simulink model "SeparateMotorModel"  (R2015b)
settings: Solver=VariableStepAuto  StartTime=0.0  StopTime=10.0  RelTol=1e-3
undefined symbols (not defined in the file): Initial, Motor, Uav
libraries: QuaternionLibrary x1, simulink_extras x1
settings Model: Creator=jban039  LastModifiedBy=jban039

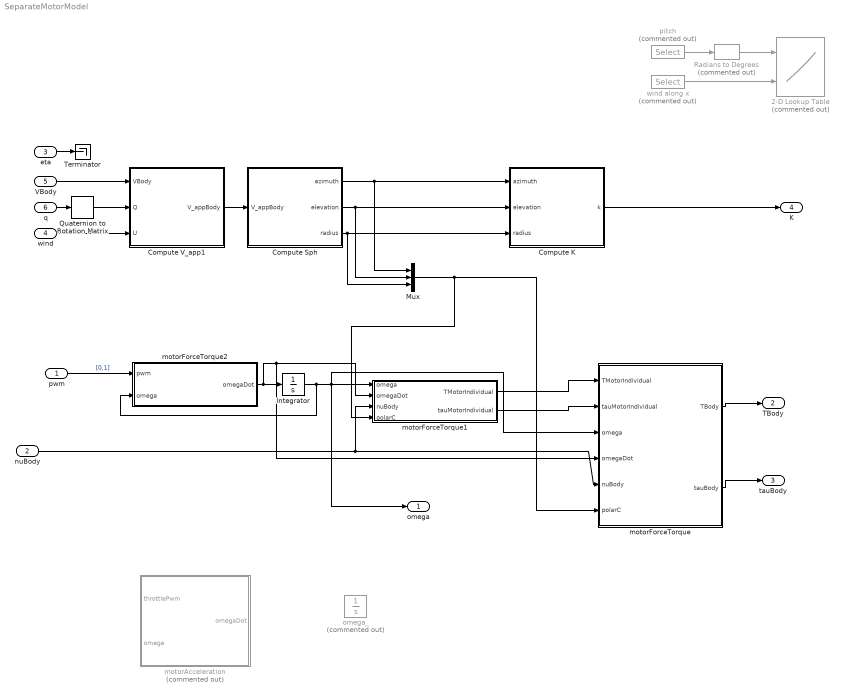
== system SeparateMotorModel ==
  pwm : Inport  PortDimensions=Uav.N_ROTORS
  nuBody : Inport  Port=2
  eta : Inport  Port=3  PortDimensions=3
  wind : Inport  Port=4  PortDimensions=3
  VBody : Inport  Port=5  PortDimensions=3
  q : Inport  Port=6  PortDimensions=4
  2-D Lookup Table : Lookup_n-D  Commented=on  BreakpointsForDimension1=[0,2.890909,6.009259676377,9.296238414,12.27875]  BreakpointsForDimension2=[0,10,20]  Table=reshape([9.55641004221352e-06,1.00990801427108e-05,1.28091919414946e-05,1.45562427543497e-05,1.63017404112369e-05,1.00884339028815e-05,1.06718323589317e-05,1.12577089455794e-05,1.21229824131359e-05,1.24606394544993e-05,9.47230336229989e-06,9.71233115660863e-06,9.65341998978562e-06,9.60249125674676e-06,8.92828582195144e-06],5,3)  InternalRulePriority=Speed  RndMeth=Simplest  InputSameDT=on
  Compute K : MATLAB Function  TreatAsAtomicUnit=on
  Compute Sph : MATLAB Function  TreatAsAtomicUnit=on
  Compute V_app1 : MATLAB Function  TreatAsAtomicUnit=on
  Integrator : Integrator
  Mux : Mux  Inputs=3
  Quaternion to Rotation Matrix : QuaternionLibrary/Quaternion to Rotation Matrix
  Radians to Degrees : simulink_extras/Transformations/Radians to Degrees  Commented=on
  Terminator : Terminator
  motorAcceleration : MATLAB Function  Commented=on  TreatAsAtomicUnit=on
  motorForceTorque : MATLAB Function  TreatAsAtomicUnit=on
  motorForceTorque1 : MATLAB Function  TreatAsAtomicUnit=on
  motorForceTorque2 : MATLAB Function  TreatAsAtomicUnit=on
  omega_ : Integrator  Commented=on  InitialCondition=Initial.OMEGA
  pitch : Selector  Commented=on  InputPortWidth=3  IndexOptions=Index vector (dialog)  Indices=[2]  OutputSizes=1
  wind along x : Selector  Commented=on  InputPortWidth=3  IndexOptions=Index vector (dialog)  Indices=[1]  OutputSizes=1
  omega : Outport
  TBody : Outport  Port=2
  tauBody : Outport  Port=3
  K : Outport  Port=4
  wires:
  motorForceTorque/2(tauBody) -> tauBody/1
  motorForceTorque/1(TBody) -> TBody/1
  pwm/1 -> motorForceTorque2/1(pwm)  "[0,1]"
  wind along x/1 -> 2-D Lookup Table/2
  pitch/1 -> Radians to Degrees/1
  Compute K/1(k) -> K/1
  Radians to Degrees/1 -> 2-D Lookup Table/1
  Quaternion to Rotation Matrix/1 -> Compute V_app1/2(Q)
  eta/1 -> Terminator/1
  wind/1 -> Compute V_app1/3(U)
  VBody/1 -> Compute V_app1/1(VBody)
  q/1 -> Quaternion to Rotation Matrix/1
  Compute V_app1/1(V_appBody) -> Compute Sph/1(V_appBody)
  Compute Sph/3(radius) -> Mux/3, Compute K/3(radius)
  Compute Sph/1(azimuth) -> Mux/1, Compute K/1(azimuth)
  Compute Sph/2(elevation) -> Mux/2, Compute K/2(elevation)
  Mux/1 -> motorForceTorque1/4(polarC), motorForceTorque/6(polarC)
  motorForceTorque1/1(TMotorIndividual) -> motorForceTorque/1(TMotorIndividual)
  motorForceTorque1/2(tauMotorIndividual) -> motorForceTorque/2(tauMotorIndividual)
  motorForceTorque2/1(omegaDot) -> motorForceTorque/4(omegaDot), motorForceTorque1/2(omegaDot), Integrator/1
  Integrator/1 -> omega/1, motorForceTorque/3(omega), motorForceTorque1/1(omega), motorForceTorque2/2(omega)
  nuBody/1 -> motorForceTorque/5(nuBody), motorForceTorque1/3(nuBody)

== matlab function SeparateMotorModel/Compute Sph ==
  data: V_appBody input; azimuth output; elevation output; radius output
function [azimuth, elevation, radius] = computeSph(V_appBody)
%#codegen

% Convert from polar to spherical coordinates
[ azimuth, elevation, radius ] = cart2sph( V_appBody(1), V_appBody(2), V_appBody(3) );

== matlab function SeparateMotorModel/Compute K ==
  data: azimuth input; k output; elevation input; radius input
function k  = computeK( azimuth, elevation, radius )
%#codegen

% Margin to prevent shattering - doesn't seem to work
% for i = 1:3
%     if ( ( V_appBody(i) > -0.002 ) && ( V_appBody(i) < 0.002 ) )
%         V_appBody(i) = 0;
%     end
% end

% % Convert from polar to spherical coordinates
% [ azimuth, elevation, radius ] = cart2sph( V_appBody(1), V_appBody(2), V_appBody(3) );

elevation = abs(elevation);

if ( elevation < 0 )
    elevation = 0;
elseif ( elevation > pi/4 )
    elevation = pi/4;
end

% if ( ( elevation < 0 ) || ( radius < 0.02 ) ) %  || ( abs( azimuth ) > pi / 4 )
%     k = 9.20186997424055e-06;
% else
k =  9.20186997424055e-06 + ...
     4.85267548640599e-06 * elevation + ...
     5.76685430140641e-07 * radius  + ...
    -8.78213951736416e-06 * elevation .^ 2 +...
    -1.77642149547229e-06 * elevation * radius + ...
    -1.52971221787416e-09 * radius^2;

k = 7.59588e-6;

% if ( k < 9.20186997424055e-06 )
%     k = 9.20186997424055e-06;
% end
% end

== matlab function SeparateMotorModel/Compute V_app1 ==
  data: VBody input; Q input; V_appBody output; U input size=3
function V_appBody = computeV_appBody(VBody, Q, U)
%#codegen

% Rotation matrix from Wind frame to Inertial frame 
R_U = [1, 0,  0;
       0, 1,  0;
       0, 0, -1];

V_appBody = VBody + Q'*R_U*U;

== matlab function SeparateMotorModel/motorForceTorque1 ==
  data: omega input; TMotorIndividual output size=[3 4]; omegaDot input; nuBody input size=3; Motor parameter; Uav parameter; tauMotorIndividual output size=[3 4]; polarC input
function [TMotorIndividual, tauMotorIndividual] = motorForceTorque(...
    omega, omegaDot, nuBody, Motor, Uav, polarC)
%#codegen

elevation = polarC(2);
windSpeed = polarC(3);

% Make assertions to avoid code generation errors
assert(Uav.N_ROTORS < 16);

%% Thrust and differential torque

% Concatenated motor force/torque vectors in respective motor frame
% eg. TMotor = [TMotor1, TMotor2, ..., TMotorN]
% where: - N is the number of rotors
%        - TMotorx (x ∈ [1,2,...,N]) is the thrust generated by motor x in
%          its own frame of reference
% TMotorIndividual = [ zeros(2, Uav.N_ROTORS);
%                      K * (omega'.^2) ];
K1 = 6.543988868292138e-05+...
    1.886359198743874e-06*sin(elevation)+...
    -7.693938774360465e-07*windSpeed+...
    2.639630950517221e-06*sin(elevation)*windSpeed+...
    2.126334444415667e-08*windSpeed^2;
K2 = -1.903771811601254e-04+...
    2.812570127999989e-03*sin(elevation)+...
    1.418616236881443e-03*windSpeed+...
    -4.525882966383329e-03*sin(elevation)*windSpeed+...
    -1.658875316836167e-05*windSpeed^2;
TMotorIndividual = [ zeros(2, Uav.N_ROTORS);
                     0.25 * 0.5 * Uav.RHO_AIR * K1 * (omega'.^2) + 0.25 * 0.5 * Uav.RHO_AIR * K2 * (omega') ]; % RECOMPUTE THRUST COEFFICIENTS AS CURRENT VALUES OUT BY FACTOR OF 4
tauMotorIndividual = [ zeros(2, Uav.N_ROTORS);
                      -Uav.ROTOR_DIRECTION .* ...
                 ( Motor.B*(omega'.^2) + Motor.I_R(3,3)*omegaDot' ) ];

== matlab function SeparateMotorModel/motorForceTorque2 ==
  data: pwm input; omegaDot output; omega input
function omegaDot  = motorForceTorque( pwm, omega)
%#codegen
rotorTimeConst = 7.006512E-02;
omegaRef = 7.969173e-1*(1000*pwm+1000)-6.528579e2;
omegaDot = (omegaRef-omega)/rotorTimeConst;

== matlab function SeparateMotorModel/motorForceTorque ==
  data: TMotorIndividual input; TBody output size=3; tauMotorIndividual input; tauBody output size=3; omega input; omegaDot input; nuBody input; Motor parameter; Uav parameter; polarC input
function [TBody, tauBody] = motorForceTorque( TMotorIndividual,tauMotorIndividual,  ...
    omega, omegaDot, nuBody, Motor, Uav, polarC)
%#codegen
assert(Uav.N_ROTORS < 16);


% Initialise matrices to store motor force/torque vectors in body frame
TBodyIndividual   = zeros(3, Uav.N_ROTORS);
tauBodyIndividual = zeros(3, Uav.N_ROTORS);

% Calculate forces and moments from each motor in the body frame
for i = 1:Uav.N_ROTORS
    l = Uav.L(i);
    beta = Uav.BETA(i);
    
    % Matrix to compute torque applied by rotor thrust
 	L = [ 0,            0,            l*sin(beta);
          0,            0,           -l*cos(beta);
         -l*sin(beta),  l*cos(beta),  0 ];

	% Motor force/torque vectors in body frame
	TBodyIndividual(:,i) = Uav.R_MOTOR_TO_BODY(:,:,i) * ...
        TMotorIndividual(:,i);
	tauBodyIndividual(:,i) = Uav.R_MOTOR_TO_BODY(:,:,i) * ...
        tauMotorIndividual(:,i) + L * TBodyIndividual(:,i);
end

%% Gyroscopic moments

% Concatenated gyroscopic moments for each rotor
M_GBodyIndividual = zeros(3, Uav.N_ROTORS);

% Concatenated motor speeds in their respective frames
omegaMotor = [ zeros(2, Uav.N_ROTORS);
               Uav.ROTOR_DIRECTION .* omega' ];

% Angular momentum in motor frame
H_MMotorSeparate = Motor.I_R * omegaMotor;

% Gyroscopic moment vectors in body frame
for i = 1:Uav.N_ROTORS
	M_GBodyIndividual(:,i) = cross( nuBody, ...
        Uav.R_MOTOR_TO_BODY(:,:,i) * H_MMotorSeparate(:,i) );
end

M_GBody = sum(M_GBodyIndividual, 2);

%% Total torque and moment

% Total force/torque in body frame
TBody = sum(TBodyIndividual, 2);
tauBody = sum(tauBodyIndividual, 2) - M_GBody;

end

== matlab function SeparateMotorModel/motorAcceleration ==
  data: throttlePwm input; omegaDot output double size=4; omega input; Motor parameter; Uav parameter
function omegaDot = motorAcceleration(throttlePwm, omega, Motor, Uav)
%#codegen

voltage = throttlePwm * Uav.NOMINAL_BATTERY_VOLTAGE;

% Motor current ignoring inductance
current = (voltage - Motor.K_E*omega) / Motor.R;

netTorque = (Motor.K_T * current) - (Motor.B * omega.^2);

% Motor angular acceleration
omegaDot = netTorque / Motor.I_R(3,3);
